simulink model "antenna_regolato"  (Simulink 7.7)
settings: Solver=ode45  StartTime=0.0  StopTime=10.0  RelTol=1e-9  AbsTol=1e-9
values from neighbouring files (symbols this model uses):
  A = [0 1; 0 -h/J]    [antenna.m]    (also in produzione.m = [0 (1-alpha)*(1-beta2); 1-beta1 0]; serbatoi.m = [-d1 0; d1 -d2])
  b = [0; 1/J]    [antenna.m]    (also in produzione.m = [1; 0]; serbatoi.m = [1; 0])
  c = [1 0]    [antenna.m]    (also in produzione.m = [0 alpha*(1-beta2)]; serbatoi.m = [0 d2])
  d = 0    [antenna.m]    (also in produzione.m; serbatoi.m)
  k = [k1 k2]    [antenna.m]    (also in motore.m; produzione.m = [k1 k2 k3]; serbatoi.m)
  l = [l1; l2]    [antenna.m]    (also in motore.m; produzione.m = [l1; l2; l3]; serbatoi.m)
  x0 = [-0.5 0]'    [antenna.m]    (also in produzione.m = [1 0]'; serbatoi.m = [1 0]')
  xcap0 = [0 0]'    [antenna.m]    (also in produzione.m; serbatoi.m)
  y0 = 0.5    [antenna.m]    (also in motore.m = 5; produzione.m = 50; serbatoi.m = 5)
settings Model: Creator=fabio  LastModifiedBy=fabio

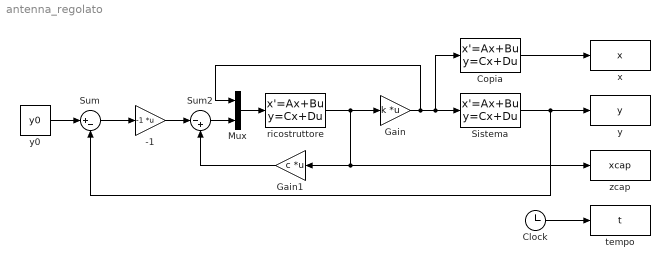
== system antenna_regolato ==
  -1 : Gain  Gain=-1  Multiplication=Matrix(K*u)
  Clock : Clock
      settings: Decimation=10
  Copia : StateSpace  A=A  B=b  C=[1 0; 0 1]  D=[0; 0]  X0=x0
  Gain : Gain  Gain=k  Multiplication=Matrix(K*u)
  Gain1 : Gain  Gain=c  Multiplication=Matrix(K*u)
  Mux : Mux  Inputs=2
  Sistema : StateSpace  A=A  B=b  C=c  D=d  X0=x0
  Sum : Sum  Inputs=|+-
  Sum2 : Sum  Inputs=|-+
  ricostruttore : StateSpace  A=A  B=[b l]  C=[1 0;0 1]  D=[0 0; 0 0]  X0=xcap0
  tempo : ToWorkspace  VariableName=t  SampleTime=-1  SaveFormat=Array
  x : ToWorkspace  VariableName=x  SampleTime=-1  SaveFormat=Array
  y : ToWorkspace  VariableName=y  SampleTime=-1  SaveFormat=Array
  y0 : Constant  Value=y0
  zcap : ToWorkspace  VariableName=xcap  SampleTime=-1  SaveFormat=Array
  wires:
  Sistema/1 -> y/1, Sum/2
  y0/1 -> Sum/1
  ricostruttore/1 -> Gain/1, zcap/1, Gain1/1
  Gain/1 -> Mux/1, Sistema/1, Copia/1
  Mux/1 -> ricostruttore/1
  Clock/1 -> tempo/1
  -1/1 -> Sum2/1
  Sum2/1 -> Mux/2
  Sum/1 -> -1/1
  Copia/1 -> x/1
  Gain1/1 -> Sum2/2
